simulink model "modelo_completo_fuzzy"  (R2017b)
settings: Solver=VariableStepAuto  StartTime=0.0  StopTime=5  RelTol=1e-3
libraries: simulink x5
settings Model: Creator=jorgeluis  LastModifiedBy=jorgeluis

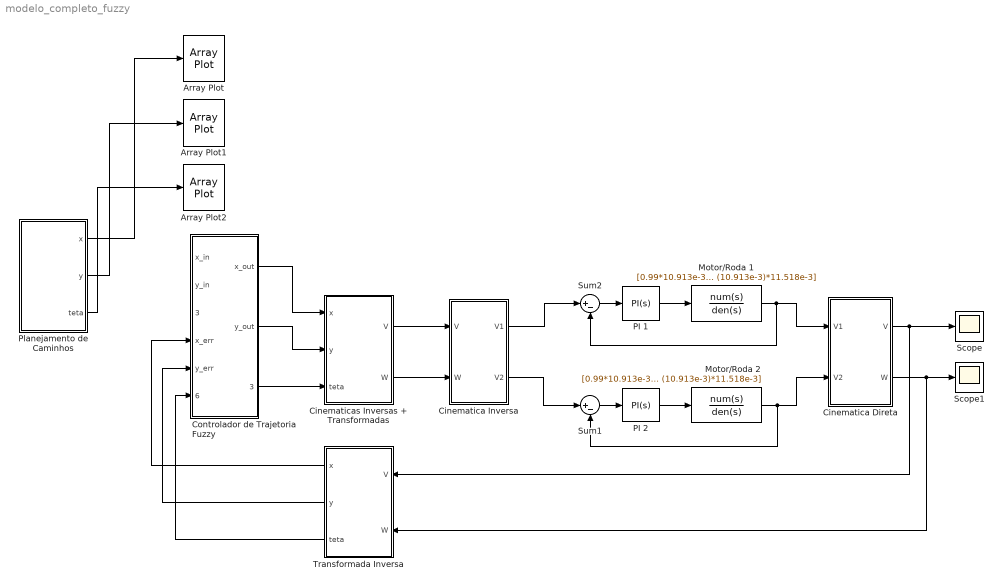
== system modelo_completo_fuzzy ==
  Array Plot : ArrayPlot
  Array Plot1 : ArrayPlot
  Array Plot2 : ArrayPlot
  Cinematica Direta : Subsystem
  Cinematica Inversa : Subsystem
  Cinematicas Inversas + Transformadas : Subsystem
  Controlador de Trajetoria Fuzzy : Subsystem
  Motor/Roda 1 : TransferFcn  Numerator=[0.99*10.913e-3]  Denominator=[(1.5506*9.35604e-3) (10.913e-3)*11.518e-3]
  Motor/Roda 2 : TransferFcn  Numerator=[0.99*10.913e-3]  Denominator=[(1.5506*9.35604e-3) (10.913e-3)*11.518e-3]
  PI 1 : simulink/Continuous/PID Controller  Controller=PI  TimeDomain=Continuous-time  SampleTime=-1  IntegratorMethod=Forward Euler  FilterMethod=Forward Euler  Form=Ideal  UseFilter=on  ControllerParametersSource=internal  P=1.0800  I=0.0433  D=0  N=0  InitialConditionSource=internal  InitialConditionForIntegrator=0  InitialConditionForFilter=0  ExternalReset=none  LimitOutput=off  UpperSaturationLimit=inf  LowerSaturationLimit=-inf  LinearizeAsGain=on  AntiWindupMode=none  Kb=1  TrackingMode=off  Kt=1  PParamMin=[]  PParamMax=[]  IParamMin=[]  IParamMax=[]  DParamMin=[]  DParamMax=[]  NParamMin=[]  NParamMax=[]  KbParamMin=[]  KbParamMax=[]  KtParamMin=[]  KtParamMax=[]  POutMin=[]  POutMax=[]  IOutMin=[]  IOutMax=[]  DOutMin=[]  DOutMax=[]  NOutMin=[]  NOutMax=[]  KbOutMin=[]  KbOutMax=[]  KtOutMin=[]  KtOutMax=[]  IntegratorOutMin=[]  IntegratorOutMax=[]  FilterOutMin=[]  FilterOutMax=[]  SumOutMin=[]  SumOutMax=[]  SumI1OutMin=[]  SumI1OutMax=[]  SumI2OutMin=[]  SumI2OutMax=[]  SumI3OutMin=[]  SumI3OutMax=[]  SumDOutMin=[]  SumDOutMax=[]  SaturationOutMin=[]  SaturationOutMax=[]  IntegratorContinuousStateAttributes=''  IntegratorStateMustResolveToSignalObject=off  IntegratorRTWStateStorageClass=Auto  FilterContinuousStateAttributes=''  FilterStateMustResolveToSignalObject=off  FilterRTWStateStorageClass=Auto  DifferentiatorICPrevScaledInput=0  DifferentiatorOutMin=[]  DifferentiatorOutMax=[]  InitialConditionSetting=State (most efficient)  FilterDiffOutCoefMin=[]  FilterDiffOutCoefMax=[]  SumDenOutMin=[]  SumDenOutMax=[]  SumNumOutMin=[]  SumNumOutMax=[]  ReciprocalOutMin=[]  ReciprocalOutMax=[]  DivideOutMin=[]  DivideOutMax=[]  TunerSelectOption=Transfer Function Based (PID Tuner App)
  PI 2 : simulink/Continuous/PID Controller  Controller=PI  TimeDomain=Continuous-time  SampleTime=-1  IntegratorMethod=Forward Euler  FilterMethod=Forward Euler  Form=Ideal  UseFilter=on  ControllerParametersSource=internal  P=1.0800  I=0.0433  D=0  N=0  InitialConditionSource=internal  InitialConditionForIntegrator=0  InitialConditionForFilter=0  ExternalReset=none  LimitOutput=off  UpperSaturationLimit=inf  LowerSaturationLimit=-inf  LinearizeAsGain=on  AntiWindupMode=none  Kb=1  TrackingMode=off  Kt=1  PParamMin=[]  PParamMax=[]  IParamMin=[]  IParamMax=[]  DParamMin=[]  DParamMax=[]  NParamMin=[]  NParamMax=[]  KbParamMin=[]  KbParamMax=[]  KtParamMin=[]  KtParamMax=[]  POutMin=[]  POutMax=[]  IOutMin=[]  IOutMax=[]  DOutMin=[]  DOutMax=[]  NOutMin=[]  NOutMax=[]  KbOutMin=[]  KbOutMax=[]  KtOutMin=[]  KtOutMax=[]  IntegratorOutMin=[]  IntegratorOutMax=[]  FilterOutMin=[]  FilterOutMax=[]  SumOutMin=[]  SumOutMax=[]  SumI1OutMin=[]  SumI1OutMax=[]  SumI2OutMin=[]  SumI2OutMax=[]  SumI3OutMin=[]  SumI3OutMax=[]  SumDOutMin=[]  SumDOutMax=[]  SaturationOutMin=[]  SaturationOutMax=[]  IntegratorContinuousStateAttributes=''  IntegratorStateMustResolveToSignalObject=off  IntegratorRTWStateStorageClass=Auto  FilterContinuousStateAttributes=''  FilterStateMustResolveToSignalObject=off  FilterRTWStateStorageClass=Auto  DifferentiatorICPrevScaledInput=0  DifferentiatorOutMin=[]  DifferentiatorOutMax=[]  InitialConditionSetting=State (most efficient)  FilterDiffOutCoefMin=[]  FilterDiffOutCoefMax=[]  SumDenOutMin=[]  SumDenOutMax=[]  SumNumOutMin=[]  SumNumOutMax=[]  ReciprocalOutMin=[]  ReciprocalOutMax=[]  DivideOutMin=[]  DivideOutMax=[]  TunerSelectOption=Transfer Function Based (PID Tuner App)
  Planejamento de Caminhos : Subsystem
  Scope : Scope
  Scope1 : Scope
  Sum1 : Sum  Inputs=|+-
  Sum2 : Sum  Inputs=|+-
  Transformada Inversa : Subsystem
  wires:
  Sum1/1 -> PI 2/1
  PI 2/1 -> Motor/Roda 2/1
  PI 1/1 -> Motor/Roda 1/1
  Sum2/1 -> PI 1/1
  Cinematica Inversa/1(V1) -> Sum2/1
  Cinematica Inversa/2(V2) -> Sum1/1
  Motor/Roda 1/1 -> Sum2/2, Cinematica Direta/1(V1)
  Motor/Roda 2/1 -> Sum1/2, Cinematica Direta/2(V2)
  Cinematica Direta/1(V) -> Transformada Inversa/1(V), Scope/1
  Cinematica Direta/2(W) -> Transformada Inversa/2(W), Scope1/1
  Cinematicas Inversas + Transformadas/1(V) -> Cinematica Inversa/1(V)
  Cinematicas Inversas + Transformadas/2(W) -> Cinematica Inversa/2(W)
  Controlador de Trajetoria Fuzzy/1(x_out) -> Cinematicas Inversas + Transformadas/1(x)
  Controlador de Trajetoria Fuzzy/2(y_out) -> Cinematicas Inversas + Transformadas/2(y)
  Controlador de Trajetoria Fuzzy/3(teta_out) -> Cinematicas Inversas + Transformadas/3(teta)
  Transformada Inversa/1(x) -> Controlador de Trajetoria Fuzzy/4(x_err)
  Transformada Inversa/3(teta) -> Controlador de Trajetoria Fuzzy/6(teta_err)
  Transformada Inversa/2(y) -> Controlador de Trajetoria Fuzzy/5(y_err)
  Planejamento de Caminhos/1(x) -> Array Plot/1
  Planejamento de Caminhos/2(y) -> Array Plot1/1
  Planejamento de Caminhos/3(teta) -> Array Plot2/1

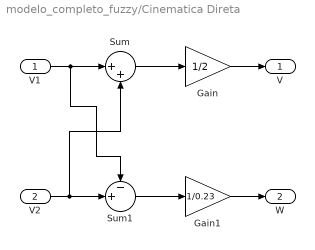
== system modelo_completo_fuzzy/Cinematica Direta ==
  V1 : Inport
  V2 : Inport  Port=2
  Gain : Gain  Gain=1/2
  Gain1 : Gain  Gain=1/0.23
  Sum : Sum  Inputs=|++
  Sum1 : Sum  Inputs=-+|
  V : Outport
  W : Outport  Port=2
  wires:
  V2/1 -> Sum/2, Sum1/2
  V1/1 -> Sum1/1, Sum/1
  Sum/1 -> Gain/1
  Gain1/1 -> W/1
  Gain/1 -> V/1
  Sum1/1 -> Gain1/1

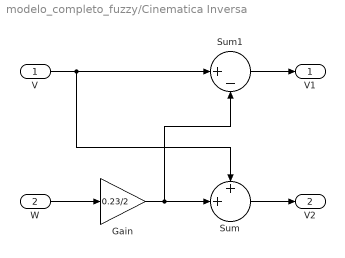
== system modelo_completo_fuzzy/Cinematica Inversa ==
  V : Inport
  W : Inport  Port=2
  Gain : Gain  Gain=0.23/2
  Sum : Sum  Inputs=++|
  Sum1 : Sum  Inputs=|+-
  V1 : Outport
  V2 : Outport  Port=2
  wires:
  W/1 -> Gain/1
  Sum1/1 -> V1/1
  Gain/1 -> Sum1/2, Sum/2
  V/1 -> Sum/1, Sum1/1
  Sum/1 -> V2/1

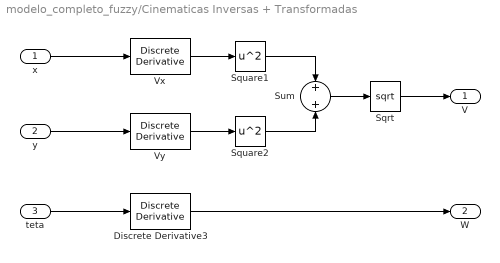
== system modelo_completo_fuzzy/Cinematicas Inversas + Transformadas ==
  x : Inport
  y : Inport  Port=2
  teta : Inport  Port=3
  Discrete Derivative3 : simulink/Discrete/Discrete Derivative  gainval=1.0  ICPrevScaledInput=0.0  OutMin=[]  OutMax=[]  OutDataType=fixdt(1, 16)  OutScaling=2^-10  DoSatur=off
  Sqrt : Sqrt  SaturateOnIntegerOverflow=on
  Square1 : Math  Operator=square  RndMeth=Zero  SaturateOnIntegerOverflow=on
  Square2 : Math  Operator=square  RndMeth=Zero  SaturateOnIntegerOverflow=on
  Sum : Sum  Inputs=+|+
  Vx : simulink/Discrete/Discrete Derivative  gainval=1.0  ICPrevScaledInput=0.0  OutMin=[]  OutMax=[]  OutDataType=fixdt(1, 16)  OutScaling=2^-10  DoSatur=off
  Vy : simulink/Discrete/Discrete Derivative  gainval=1.0  ICPrevScaledInput=0.0  OutMin=[]  OutMax=[]  OutDataType=fixdt(1, 16)  OutScaling=2^-10  DoSatur=off
  V : Outport
  W : Outport  Port=2
  wires:
  Discrete Derivative3/1 -> W/1
  teta/1 -> Discrete Derivative3/1
  x/1 -> Vx/1
  Sqrt/1 -> V/1
  y/1 -> Vy/1
  Vx/1 -> Square1/1
  Vy/1 -> Square2/1
  Square1/1 -> Sum/1
  Square2/1 -> Sum/2
  Sum/1 -> Sqrt/1

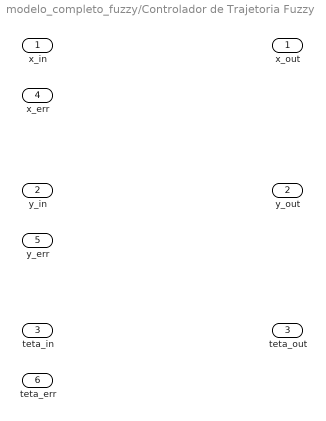
== system modelo_completo_fuzzy/Controlador de Trajetoria Fuzzy ==
  x_in : Inport
  y_in : Inport  Port=2
  teta_in : Inport  Port=3
  x_err : Inport  Port=4
  y_err : Inport  Port=5
  teta_err : Inport  Port=6
  x_out : Outport
  y_out : Outport  Port=2
  teta_out : Outport  Port=3

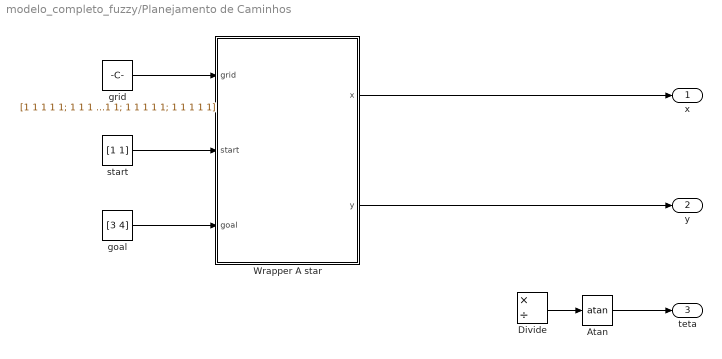
== system modelo_completo_fuzzy/Planejamento de Caminhos ==
  Atan : Trigonometry  Operator=atan
  Divide : Product  Inputs=*/
  Wrapper A star : MATLAB Function  TreatAsAtomicUnit=on
  goal : Constant  Value=[3 4]  OutDataTypeStr=Inherit: Inherit via back propagation
  grid : Constant  Value=[1 1 1 1 1; 1 1 1 1 1; 1 1 1 1 1; 1 1 1 1 1; 1 1 1 1 1]  OutDataTypeStr=Inherit: Inherit via back propagation
  start : Constant  Value=[1 1]  OutDataTypeStr=Inherit: Inherit via back propagation
  x : Outport
  y : Outport  Port=2
  teta : Outport  Port=3
  wires:
  Wrapper A star/1(x) -> x/1
  Wrapper A star/2(y) -> y/1
  Atan/1 -> teta/1
  grid/1 -> Wrapper A star/1(grid)
  Divide/1 -> Atan/1
  start/1 -> Wrapper A star/2(start)
  goal/1 -> Wrapper A star/3(goal)

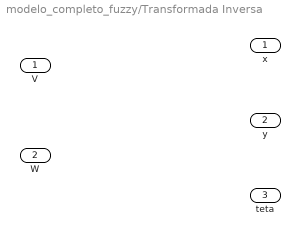
== system modelo_completo_fuzzy/Transformada Inversa ==
  V : Inport
  W : Inport  Port=2
  x : Outport
  y : Outport  Port=2
  teta : Outport  Port=3

== matlab function modelo_completo_fuzzy/Planejamento de Caminhos/Wrapper A star ==
  data: grid input; start input; x output size=[1 20]; goal input; y output
% Autores: Jorgeluis Guerra
%          Luis Braga
%          Saulo Alves

% Funcao wrapper que insere o algoritmo do A estrela dentro do modelo do
% robo

function [x,y] = wrapper_a_star(grid, start, goal)

   % Valor 'infinito'
   INF = 100000;
   % Limites do grid de celulas
   GRID_MIN = 1;
   GRID_MAX = 5;

   start_node.x = start(1);
   start_node.y = start(2);
   start_node.g = INF;
   start_node.f = INF;
   start_node.camefrom = [];

   goal_node.x = goal(1);
   goal_node.y = goal(2);
   goal_node.g = INF;
   goal_node.f = INF;
   goal_node.camefrom = [];

   path_nodes = a_star(start_node, goal_node);

   x = zeros(1,20);
   y = zeros(1,20);
   j = 1;
   for i = path_nodes
      x(j) = i.x;
      y(j) = i.y;
      j = j + 1;
   end
end
